simulink model "Rectifier_AND_Buck_Converter"  (R2015a)
settings: Solver=ode45  StartTime=0.0  StopTime=0.01  RelTol=1e-3
values from neighbouring files (symbols this model uses):
  C = 19.5e-06    (= 1.95e-05)    [RECTIFIER_AND_BUCK_CONVERTER_Script.m]
  D = 12/380    (= 0.0315789473684)    [RECTIFIER_AND_BUCK_CONVERTER_Script.m]
  fs = 400e03    (= 400000)    [RECTIFIER_AND_BUCK_CONVERTER_Script.m]
  L = 12.12e-06    (= 1.212e-05)    [RECTIFIER_AND_BUCK_CONVERTER_Script.m]
  RL = 5    [RECTIFIER_AND_BUCK_CONVERTER_Script.m]
settings Model: Creator=Koustubh  LastModifiedBy=Koustubh

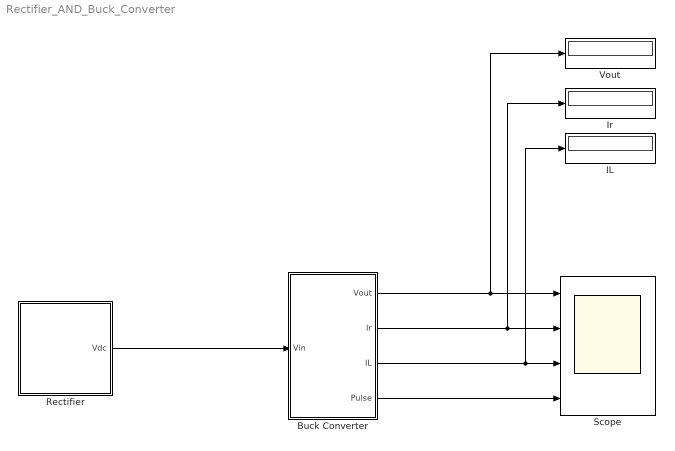
== system Rectifier_AND_Buck_Converter ==
  Buck Converter : Subsystem
  IL : Display
  Ir : Display
  Rectifier : Subsystem
  Scope : Scope  NumInputPorts=4
      settings: YMin=-5~-5~-5~-5  YMax=5~5~5~5  SaveName=ScopeData2
  Vout : Display
  wires:
  Rectifier/1(Vdc) -> Buck Converter/1(Vin)
  Buck Converter/1(Vout) -> Vout/1, Scope/1
  Buck Converter/2(Ir) -> Ir/1, Scope/2
  Buck Converter/3(IL) -> IL/1, Scope/3
  Buck Converter/4(Pulse) -> Scope/4

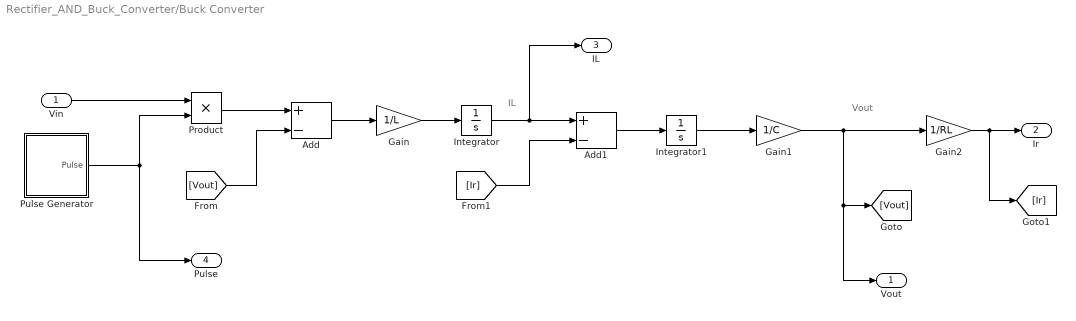
== system Rectifier_AND_Buck_Converter/Buck Converter ==
  note: Vout
  note: IL
  Vin : Inport
  Add : Sum  Inputs=+-
  Add1 : Sum  Inputs=+-
  Gain : Gain  Gain=1/L
  Gain1 : Gain  Gain=1/C
  Gain2 : Gain  Gain=1/RL
  Integrator : Integrator
  Integrator1 : Integrator
  Product : Product
  Pulse Generator : Subsystem
  Vout : Outport
  Ir : Outport  Port=2
  IL : Outport  Port=3
  Pulse : Outport  Port=4
  wires:
  Vin/1 -> Product/1
  Pulse Generator/1(Pulse) -> Pulse/1, Product/2
  Product/1 -> Add/1
  [Vout] -> Add/2
  Add/1 -> Gain/1
  Gain/1 -> Integrator/1
  Integrator/1 -> IL/1, Add1/1
  [Ir] -> Add1/2
  Add1/1 -> Integrator1/1
  Integrator1/1 -> Gain1/1
  Gain1/1 -> Vout/1, [Vout], Gain2/1
  Gain2/1 -> Ir/1, [Ir]

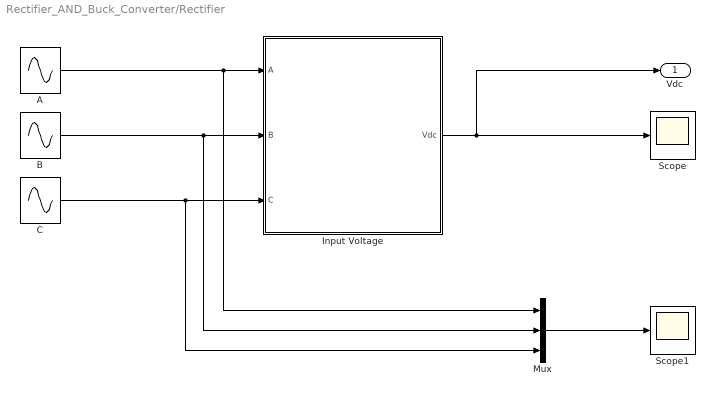
== system Rectifier_AND_Buck_Converter/Rectifier ==
  A : Sin  Amplitude=230  Frequency=2*pi*50  SampleTime=0
  B : Sin  Amplitude=230  Frequency=2*pi*50  Phase=2*pi/3  SampleTime=0
  C : Sin  Amplitude=230  Frequency=2*pi*50  Phase=4*pi/3  SampleTime=0
  Input Voltage : Subsystem
  Mux : Mux  Inputs=3
  Scope : Scope
  Scope1 : Scope
  Vdc : Outport
  wires:
  B/1 -> Mux/2, Input Voltage/2(B)
  A/1 -> Mux/1, Input Voltage/1(A)
  Input Voltage/1(Vdc) -> Vdc/1, Scope/1
  Mux/1 -> Scope1/1
  C/1 -> Mux/3, Input Voltage/3(C)

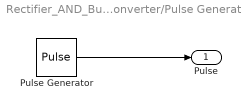
== system Rectifier_AND_Buck_Converter/Buck Converter/Pulse Generator ==
  Pulse Generator : DiscretePulseGenerator  PulseType=Time based  Period=1/fs  PulseWidth=D*100
  Pulse : Outport
  wires:
  Pulse Generator/1 -> Pulse/1

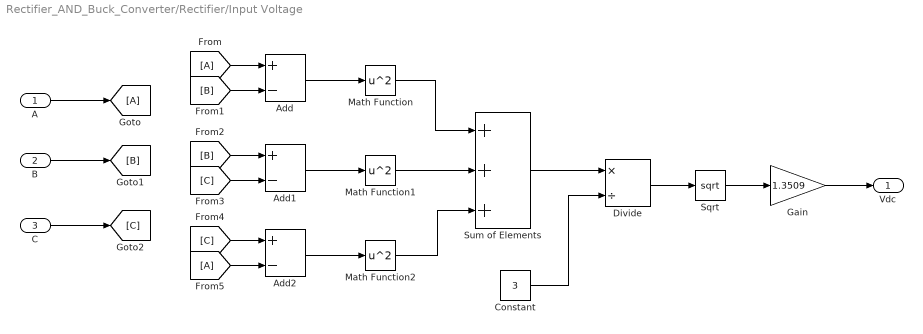
== system Rectifier_AND_Buck_Converter/Rectifier/Input Voltage ==
  A : Inport
  B : Inport  Port=2
  C : Inport  Port=3
  Add : Sum  Inputs=+-
  Add1 : Sum  Inputs=+-
  Add2 : Sum  Inputs=+-
  Constant : Constant  Value=3
  Divide : Product  Inputs=*/
  Gain : Gain  Gain=1.3509
  Math Function : Math  Operator=square  SaturateOnIntegerOverflow=on
  Math Function1 : Math  Operator=square  SaturateOnIntegerOverflow=on
  Math Function2 : Math  Operator=square  SaturateOnIntegerOverflow=on
  Sqrt : Sqrt  SaturateOnIntegerOverflow=on
  Sum of Elements : Sum  Inputs=+++
  Vdc : Outport
  wires:
  Sum of Elements/1 -> Divide/1
  Math Function/1 -> Sum of Elements/1
  Constant/1 -> Divide/2
  Divide/1 -> Sqrt/1
  Math Function1/1 -> Sum of Elements/2
  Math Function2/1 -> Sum of Elements/3
  [C] -> Add2/1
  [B] -> Add1/1
  [C] -> Add1/2
  [A] -> Add2/2
  [B] -> Add/2
  [A] -> Add/1
  A/1 -> [A]
  C/1 -> [C]
  B/1 -> [B]
  Add1/1 -> Math Function1/1
  Add2/1 -> Math Function2/1
  Add/1 -> Math Function/1
  Sqrt/1 -> Gain/1
  Gain/1 -> Vdc/1
